simulink model "flexiFlightVis_lib_example"  (R2018b)
settings: Solver=ode2  StartTime=0.0  StopTime=100  FixedStep=1/60  RelTol=1e-3
values from neighbouring files (symbols this model uses):
  fuselage_state = fuselage.state    [flexiFlightVis_lib_example_init.m]
  rigid_body = rigidBodyCreate()    [flexiFlightVis_lib_example_init.m]
  wing_1_state = wing_1.state    [flexiFlightVis_lib_example_init.m]
  wing_2_state = wing_2.state    [flexiFlightVis_lib_example_init.m]
undefined symbols (not defined in the file or in its folder): config
libraries: flexiFlightVis_lib x1
settings Model: EnablePacing=on  Creator=akuzolap  LastModifiedBy=yannic
settings DataIOCC: ReturnWorkspaceOutputs=on

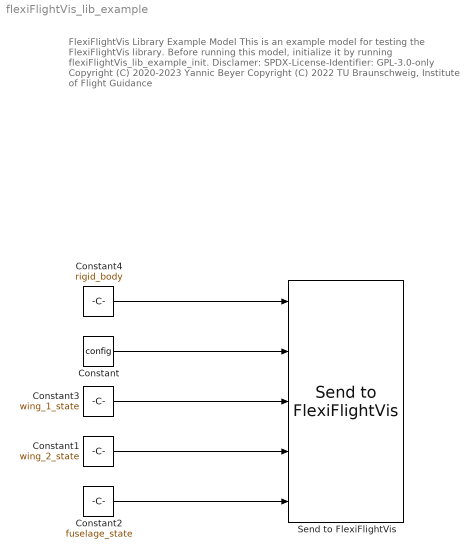
== system flexiFlightVis_lib_example ==
  note: FlexiFlightVis Library Example Model
      |
      | This is an example model for testing the FlexiFlightVis library.
      | Before running this model, initialize it by running flexiFlightVis_lib_example_init.
      |
      | Disclamer:
      | SPDX-License-Identifier: GPL-3.0-only
      |
      | Copyright (C) 2020-2023 Yannic Beyer
      | Copyright (C) 2022 TU Braunschweig, Institute of Flight Guidance
  Constant : Constant  Value=config  OutDataTypeStr=Bus: config_bus
  Constant1 : Constant  Value=wing_2_state  OutDataTypeStr=Bus: wing_2_state_bus
  Constant2 : Constant  Value=fuselage_state  OutDataTypeStr=Bus: fuselage_state_bus
  Constant3 : Constant  Value=wing_1_state  OutDataTypeStr=Bus: wing_1_state_bus
  Constant4 : Constant  Value=rigid_body  OutDataTypeStr=Bus: rigid_body_bus
  Send to FlexiFlightVis : flexiFlightVis_lib/Send to FlexiFlightVis  sample_time=1/60  ip_address='localhost'  ip_port=4321  wing_cell={wing_1.state,wing_2.state}  fuse_cell={fuselage.state}
  wires:
  Constant/1 -> Send to FlexiFlightVis/2
  Constant3/1 -> Send to FlexiFlightVis/3
  Constant4/1 -> Send to FlexiFlightVis/1
  Constant1/1 -> Send to FlexiFlightVis/4
  Constant2/1 -> Send to FlexiFlightVis/5
